simulink model "untitled1"  (R2018a)
settings: Solver=VariableStepAuto  StartTime=0.0  StopTime=100  RelTol=1e-3
settings Model: Creator=johnb  LastModifiedBy=johnb

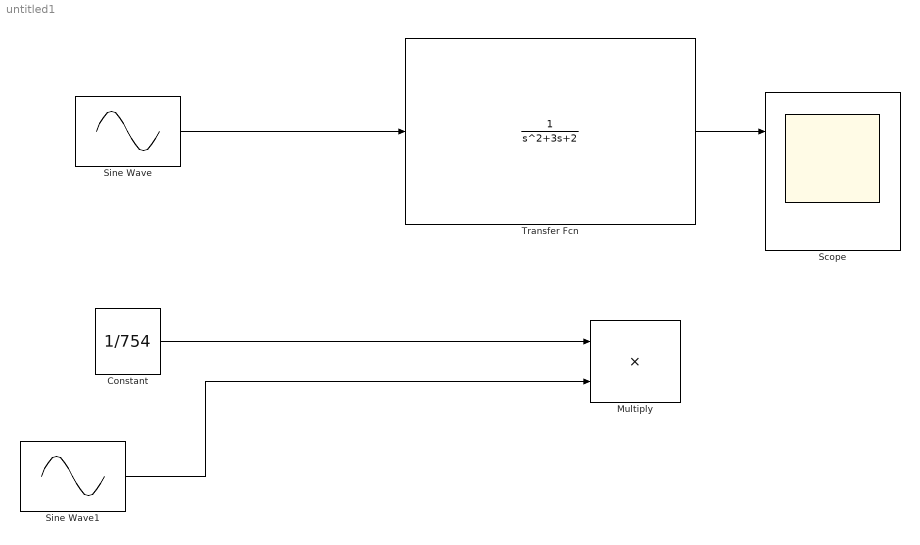
== system untitled1 ==
  Constant : Constant  Value=1/754
  Multiply : Product
  Scope : Scope  NumInputPorts=2
  Sine Wave : Sin  Amplitude=4  Frequency=5  SampleTime=0
  Sine Wave1 : Sin  Amplitude=4  Frequency=5  SampleTime=0
  Transfer Fcn : TransferFcn  Denominator=[1 3 2]
  wires:
  Sine Wave/1 -> Transfer Fcn/1
  Transfer Fcn/1 -> Scope/1
  Constant/1 -> Multiply/1
  Sine Wave1/1 -> Multiply/2
